simulink model "openloopmodel_saturation_control101"  (R2025b)
settings: Solver=VariableStepAuto  StartTime=0.0  StopTime=stoptime  RelTol=1e-3
undefined symbols (not defined in the file or in its folder): den, gain, num, target, umax, umin
settings Model: Creator=Anthony Rossiter  LastModifiedBy=Anthony Rossiter

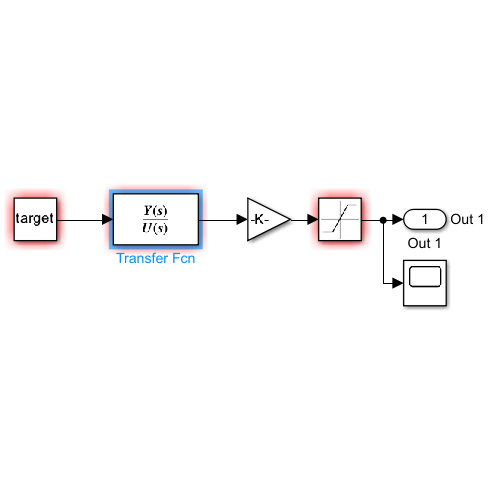
[thumbnail: Simulink's stored preview of the top-level diagram]
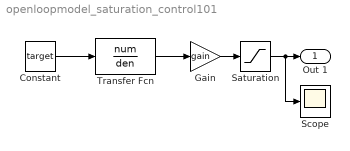
== system openloopmodel_saturation_control101 ==
  Constant : Constant  Value=target
  Gain : Gain  Gain=gain
  Saturation : Saturate  UpperLimit=umax  LowerLimit=umin
  Scope : Scope
      settings: ActiveDisplayYMinimum=-0.24999999999999994  ActiveDisplayYMaximum=2.25
  Transfer Fcn : TransferFcn  Numerator=num  Denominator=den
  Out 1 : Outport  SignalName=Out 1
  wires:
  Constant/1 -> Transfer Fcn/1
  Gain/1 -> Saturation/1
  Saturation/1 -> Scope/1, Out 1/1
  Transfer Fcn/1 -> Gain/1
